simulink model "lineFollowerModel"  (R2020a)
settings: Solver=ode4  StartTime=0.0  StopTime=20  FixedStep=0.0001  RelTol=1e-3
values from neighbouring files (symbols this model uses):
  b = -0.05    [define_constants.m]
  cRoll = 0.1    [define_constants.m]
  g = 9.81    [define_constants.m]
  I_T = 0.1    [define_constants.m]
  I_yy = 5.0000e-05    (= 5e-05)    [define_constants.m]
  K = 0.0089    [define_constants.m]
  L = 2.3E-2    (= 0.023)    [define_constants.m]
  m_T = 1 * mass_scale    [define_constants.m]
  N = 50    [define_constants.m]
  R = 2.2    [define_constants.m]
  row1 = 0.1    [define_constants.m]
  row2 = row1*wheel_ratio_scale    [define_constants.m]
  sX = row1    (= 0.1)    [define_constants.m]
  sY = 0    [define_constants.m]
  Vmax = 12    [define_constants.m]
  W = line_width/2    [define_constants.m]
settings Model: Creator=Amir  LastModifiedBy=matthewterblanche
settings SFSimCC: CustomCodeUndefinedFunction=UseInterfaceOnly

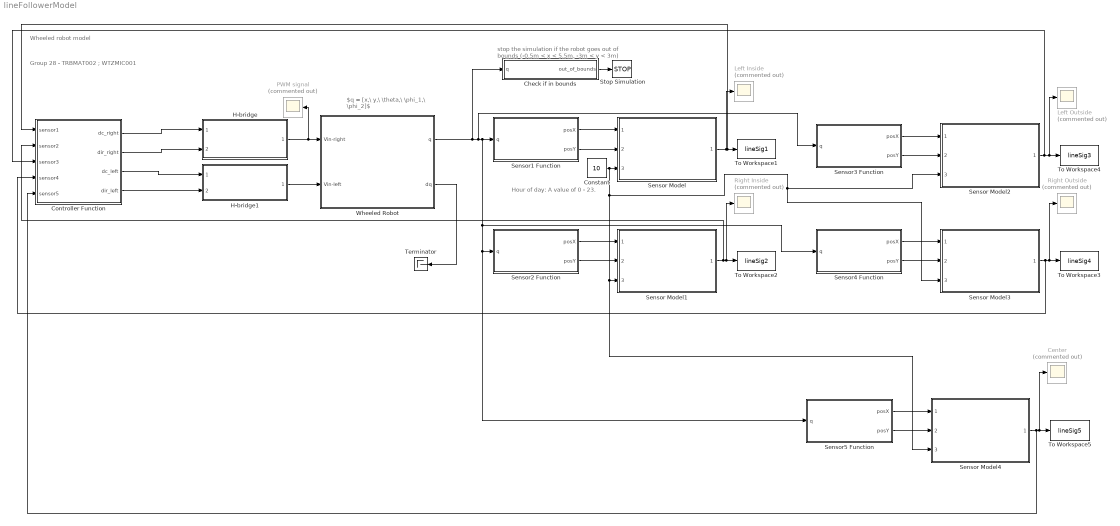
== system lineFollowerModel ==
  note: Group 28 - TRBMAT002 ; WTZMIC001
  note: Hour of day: A value of 0 - 23.
  note: Wheeled robot model
  note: $q = [x,\ y,\ \theta,\ \phi_1,\ \phi_2]$
  note: stop the simulation if the robot goes out of bounds (-0.5m < x < 5.5m, -3m < y < 3m)
  Center : Scope  Commented=on
  Check if in bounds : MATLAB Function  TreatAsAtomicUnit=on
  Constant : Constant  Value=10
  Controller Function : MATLAB Function  TreatAsAtomicUnit=on
  H-bridge : Subsystem  ReferencedSubsystem=H_bridge
  H-bridge1 : Subsystem  ReferencedSubsystem=H_bridge
  Left Inside : Scope  Commented=on
  Left Outside : Scope  Commented=on
  PWM signal : Scope  Commented=on
  Right Inside : Scope  Commented=on
  Right Outside : Scope  Commented=on
  Sensor Model{,1..4} (5 alike) : Subsystem  ReferencedSubsystem=Sensor_Model
  Sensor1 Function : MATLAB Function  TreatAsAtomicUnit=on
  Sensor2 Function : MATLAB Function  TreatAsAtomicUnit=on
  Sensor3 Function : MATLAB Function  TreatAsAtomicUnit=on
  Sensor4 Function : MATLAB Function  TreatAsAtomicUnit=on
  Sensor5 Function : MATLAB Function  TreatAsAtomicUnit=on
  Stop Simulation : Stop
  Terminator : Terminator
  To Workspace1 : ToWorkspace  VariableName=lineSig1  SampleTime=-1
  To Workspace2 : ToWorkspace  VariableName=lineSig2  SampleTime=-1
  To Workspace3 : ToWorkspace  VariableName=lineSig4  SampleTime=-1
  To Workspace4 : ToWorkspace  VariableName=lineSig3  SampleTime=-1
  To Workspace5 : ToWorkspace  VariableName=lineSig5  SampleTime=-1
  Wheeled Robot : Subsystem
  wires:
  H-bridge/1 -> Wheeled Robot/1(Vin-right), PWM signal/1
  H-bridge1/1 -> Wheeled Robot/2(Vin-left)
  Wheeled Robot/2(dq) -> Terminator/1
  Check if in bounds/1(out_of_bounds) -> Stop Simulation/1
  Sensor1 Function/2(posY) -> Sensor Model/2
  Sensor1 Function/1(posX) -> Sensor Model/1
  Sensor Model/1 -> Left Inside/1, Controller Function/1(sensor1), To Workspace1/1
  Sensor2 Function/1(posX) -> Sensor Model1/1
  Sensor2 Function/2(posY) -> Sensor Model1/2
  Sensor Model1/1 -> Controller Function/2(sensor2), Right Inside/1, To Workspace2/1
  Controller Function/1(dc_right) -> H-bridge/1
  Controller Function/2(dir_right) -> H-bridge/2
  Controller Function/3(dc_left) -> H-bridge1/1
  Controller Function/4(dir_left) -> H-bridge1/2
  Sensor4 Function/1(posX) -> Sensor Model3/1
  Sensor4 Function/2(posY) -> Sensor Model3/2
  Constant/1 -> Sensor Model/3, Sensor Model3/3, Sensor Model2/3, Sensor Model4/3, Sensor Model1/3
  Sensor Model2/1 -> Controller Function/3(sensor3), Left Outside/1, To Workspace4/1
  Sensor3 Function/1(posX) -> Sensor Model2/1
  Sensor3 Function/2(posY) -> Sensor Model2/2
  Wheeled Robot/1(q) -> Check if in bounds/1(q), Sensor3 Function/1(q), Sensor4 Function/1(q), Sensor5 Function/1(q), Sensor2 Function/1(q), Sensor1 Function/1(q)
  Sensor Model4/1 -> Controller Function/5(sensor5), Center/1, To Workspace5/1
  Sensor5 Function/1(posX) -> Sensor Model4/1
  Sensor5 Function/2(posY) -> Sensor Model4/2
  Sensor Model3/1 -> Controller Function/4(sensor4), Right Outside/1, To Workspace3/1

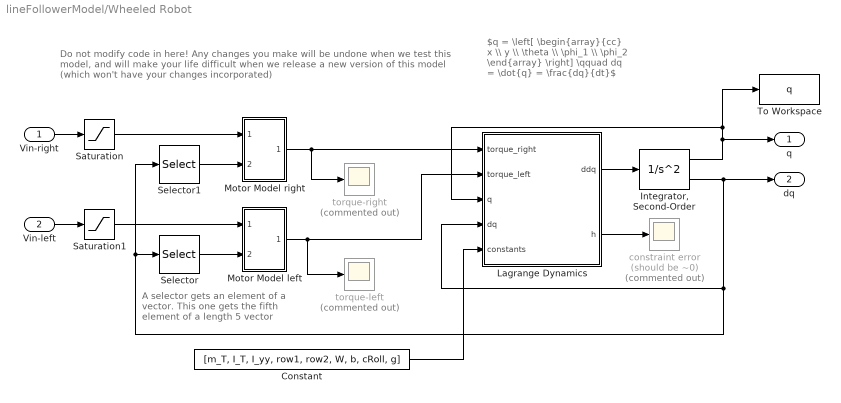
== system lineFollowerModel/Wheeled Robot ==
  note: A selector gets an element of a vector. This one gets the fifth element of a length 5 vector
  note: Do not modify code in here! Any changes you make will be undone when we test this model, and will make your life difficult when we release a new version of this model (which won't have your changes incorporated)
  note: $q = \left[ \begin{array}{cc} x \\ y \\ \theta \\ \phi_1 \\ \phi_2 \end{array} \right] \qquad dq = \dot{q} = \frac{dq}{dt}$
  Vin-right : Inport
  Vin-left : Inport  Port=2
  Constant : Constant  Value=[m_T, I_T, I_yy, row1, row2, W, b, cRoll, g]
  "Integrator, Second-Order" : SecondOrderIntegrator  ICX=[0 0 0 0 0]  ICDXDT=[0 0 0 0 0]
  Lagrange Dynamics : MATLAB Function  TreatAsAtomicUnit=on
  "Motor Model left " : Subsystem
  Motor Model right : Subsystem
  Saturation : Saturate  UpperLimit=Vmax  LowerLimit=-Vmax
  Saturation1 : Saturate  UpperLimit=Vmax  LowerLimit=-Vmax
  Selector : Selector  InputPortWidth=5  IndexOptions=Index vector (dialog)  Indices=[5]  OutputSizes=1
  Selector1 : Selector  InputPortWidth=5  IndexOptions=Index vector (dialog)  Indices=[4]  OutputSizes=1
  To Workspace : ToWorkspace  VariableName=q  SampleTime=0.01
  constraint error (should be ~0) : Scope  Commented=on
  torque-left : Scope  Commented=on
  torque-right : Scope  Commented=on
  q : Outport
  dq : Outport  Port=2
  wires:
  Selector/1 -> "Motor Model left "/2(Omega)
  Selector1/1 -> Motor Model right/2(Omega)
  Motor Model right/1(Tout) -> Lagrange Dynamics/1(torque_right), torque-right/1
  Vin-right/1 -> Saturation/1
  Vin-left/1 -> Saturation1/1
  "Integrator, Second-Order"/1 -> To Workspace/1, Lagrange Dynamics/3(q), q/1
  "Motor Model left "/1(Tout) -> Lagrange Dynamics/2(torque_left), torque-left/1
  "Integrator, Second-Order"/2 -> dq/1, Lagrange Dynamics/4(dq), Selector/1, Selector1/1
  Saturation/1 -> Motor Model right/1(Vin)
  Saturation1/1 -> "Motor Model left "/1(Vin)
  Lagrange Dynamics/1(ddq) -> "Integrator, Second-Order"/1
  Lagrange Dynamics/2(h) -> constraint error (should be ~0)/1
  Constant/1 -> Lagrange Dynamics/5(constants)

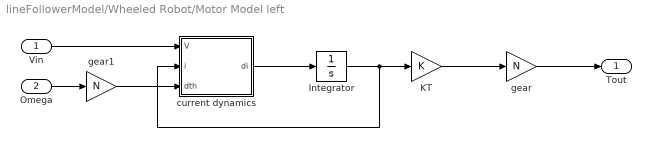
== system lineFollowerModel/Wheeled Robot/Motor Model left  ==
  Vin : Inport
  Omega : Inport  Port=2
  Integrator : Integrator
  KT : Gain  Gain=K
  current dynamics : MATLAB Function  TreatAsAtomicUnit=on
  gear : Gain  Gain=N
  gear1 : Gain  Gain=N
  Tout : Outport  VectorParamsAs1DForOutWhenUnconnected=off
  wires:
  gear1/1 -> current dynamics/3(dth)
  Integrator/1 -> current dynamics/2(i), KT/1
  Omega/1 -> gear1/1
  gear/1 -> Tout/1
  current dynamics/1(di) -> Integrator/1
  KT/1 -> gear/1
  Vin/1 -> current dynamics/1(V)

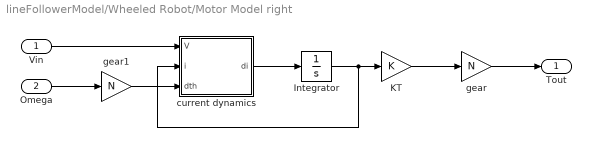
== system lineFollowerModel/Wheeled Robot/Motor Model right ==
  Vin : Inport
  Omega : Inport  Port=2
  Integrator : Integrator
  KT : Gain  Gain=K
  current dynamics : MATLAB Function  TreatAsAtomicUnit=on
  gear : Gain  Gain=N
  gear1 : Gain  Gain=N
  Tout : Outport  VectorParamsAs1DForOutWhenUnconnected=off
  wires:
  Vin/1 -> current dynamics/1(V)
  KT/1 -> gear/1
  current dynamics/1(di) -> Integrator/1
  gear/1 -> Tout/1
  Omega/1 -> gear1/1
  Integrator/1 -> current dynamics/2(i), KT/1
  gear1/1 -> current dynamics/3(dth)

== matlab function lineFollowerModel/Sensor4 Function ==
  data: posX output; q input; sY parameter; sX parameter; posY output
function [posX, posY] = sensor4Position(q, sY, sX)

x = q(1);
y = q(2);
th = q(3);


sX = 0.082;   % Sets sensor just before the front of the robot
sY = -0.082;    % Sets the sensor far right of the line. In the middle of the line and the right side of the robot

posSens_I = [x + sX*cos(th) - sY*sin(th)
    y + sY*cos(th) + sX*sin(th)];

posX = posSens_I(1);
posY = posSens_I(2);

== matlab function lineFollowerModel/Sensor3 Function ==
  data: posX output; q input; sY parameter; sX parameter; posY output
function [posX, posY] = sensor3Position(q, sY, sX)

x = q(1);
y = q(2);
th = q(3);


sX = 0.082;   % Sets sensor just before the front of the robot
sY = 0.085;    % Sets the sensor far left of the line. In the middle of the line and the left side of the robot


posSens_I = [x + sX*cos(th) - sY*sin(th)
    y + sY*cos(th) + sX*sin(th)];

posX = posSens_I(1);
posY = posSens_I(2);

== matlab function lineFollowerModel/Sensor5 Function ==
  data: posX output; q input; sY parameter; sX parameter; posY output
function [posX, posY] = sensor5Position(q, sY, sX)

x = q(1);
y = q(2);
th = q(3);


sX = 0.01;   % Sets sensor at the front of the robot
sY = 0;    % Sets the sensor at the centre of the robot

posSens_I = [x + sX*cos(th) - sY*sin(th)
    y + sY*cos(th) + sX*sin(th)];

posX = posSens_I(1);
posY = posSens_I(2);

== matlab function lineFollowerModel/Wheeled Robot/Motor Model left /current dynamics ==
  data: V input; di output; i input; L parameter; K parameter; R parameter; dth input
function di = dyn(V, i, L, K, R, dth)

di = (V-K*dth-R*i)/L;

== matlab function lineFollowerModel/Wheeled Robot/Lagrange Dynamics ==
  settings: updateMethod=DISCRETE
  data: ddq output size=5; h output size=3; torque_right input; torque_left input; q input; dq input; constants input
%% These dynamics are based on: 
% https://robotics.caltech.edu/~me72/class/DiffDrive2.pdf
% Assume 'd' is 0
function [ddq, h] = dyn(torque_right, torque_left, q, dq, constants)
m_T = constants(1);
I_T = constants(2);
I_yy = constants(3);
row1 = constants(4);
row2 = constants(5);
W = constants(6);
b = constants(7);
cRoll = constants(8);
g = constants(9);

%% Admin
% x = q(1);
% y = q(2);
th = q(3);
% phi1 = q(4);
% phi2 = q(5);

dx = dq(1);
dy = dq(2);
dth = dq(3);
dphi1 = dq(4);
dphi2 = dq(5);


%% Calculate the matrices
% Mass
M = [m_T,   0,   0,    0,    0
       0, m_T,   0,    0,    0
       0,   0, I_T,    0,    0
       0,   0,   0, I_yy,    0
       0,   0,   0,    0, I_yy];

temp = [-sin(th), cos(th), cos(th)
         cos(th), sin(th), sin(th)
               0,     W/2,    -W/2
               0,  - row1,       0
               0,       0,   -row2];

C = transpose(temp);

temp = [ -dth*cos(th), -dth*sin(th), -dth*sin(th)
         -dth*sin(th),  dth*cos(th),  dth*cos(th)
                    0,            0,            0
                    0,            0,            0
                    0,            0,            0];

dC = transpose(temp);

% Input force
T = [0; 0; 0; torque_right + b*dphi1; torque_left + b*dphi2];

% Rolling resistance
vWheel1 = (W*dth)/2 + dx*cos(th) + dy*sin(th);
vWheel2 = dx*cos(th) - (W*dth)/2 + dy*sin(th);
sgnWheel1 = sign(vWheel1);
sgnWheel2 = sign(vWheel2);

F1 = -sgnWheel1*m_T*g*cRoll;
F2 = -sgnWheel2*m_T*g*cRoll;

% input force mapping
Q =  [F1*cos(th) + F2*cos(th)
      F1*sin(th) + F2*sin(th)
          (F1*W)/2 - (F2*W)/2
                            0
                            0];

%% Calculate Lagrange Multipliers
% lambda = -inv(C*inv(M)*transpose(C))*(C*inv(M)*(T+Q) + dC*dq);
lambda = -inv(C*(M\transpose(C)))*(C*(M\(T+Q)) + dC*dq);

h = [                          dy*cos(th) - dx*sin(th)
      (W*dth)/2 - dphi1*row1 + dx*cos(th) + dy*sin(th)
      dx*cos(th) - dphi2*row2 - (W*dth)/2 + dy*sin(th)];


%% Calculate acceleration
ddq = M\(transpose(C)*lambda + T + Q);

end

== matlab function lineFollowerModel/Wheeled Robot/Motor Model right/current dynamics ==
  data: V input; di output; i input; L parameter; K parameter; R parameter; dth input
function di = dyn(V, i, L, K, R, dth)

di = (V - K*dth - R*i)/L;

== matlab function lineFollowerModel/Sensor1 Function ==
  data: posX output; q input; sY parameter; sX parameter; posY output
function [posX, posY] = sensor1Position(q, sY, sX)

x = q(1);
y = q(2);
th = q(3);

sX = 0.1;   % Sets sensor at the front of the robot
sY = 0.019;    % Sets the sensor just to the left of the line


posSens_I = [x + sX*cos(th) - sY*sin(th)
    y + sY*cos(th) + sX*sin(th)];

posX = posSens_I(1);
posY = posSens_I(2);

== matlab function lineFollowerModel/Sensor2 Function ==
  data: posX output; q input; sY parameter; sX parameter; posY output
function [posX, posY] = sensor2Position(q, sY, sX)

x = q(1);
y = q(2);
th = q(3);


sX = 0.1;   % Sets sensor at the front of the robot
sY = -0.024;    % Sets the sensor just to the right of the line

posSens_I = [x + sX*cos(th) - sY*sin(th)
    y + sY*cos(th) + sX*sin(th)];

posX = posSens_I(1);
posY = posSens_I(2);

== matlab function lineFollowerModel/Check if in bounds ==
  data: q input; out_of_bounds output
function out_of_bounds = fcn(q)
x = q(1);
y = q(2);

in_bounds = -0.5 < x && x < 5.5 && -3 < y && y < 3;

out_of_bounds = ~in_bounds;

if out_of_bounds
    disp("Stopping simulation - robot is out of bounds!")
end

== matlab function lineFollowerModel/Controller Function ==
  data: sensor1 input; dc_right output; sensor2 input; dir_right output; dc_left output; dir_left output; sensor3 input; sensor4 input; sensor5 input
function [dc_right,dir_right,dc_left,dir_left] = controller(sensor1, sensor2, sensor3, sensor4, sensor5)

% Persistent variables ensure the value is not reset after every function call

persistent moveLeft;

if isempty(moveLeft)
    moveLeft = 1;
end

persistent moveRight;


if isempty(moveRight)
    moveRight = 1;
end

persistent robotSpeed;

if isempty(robotSpeed)
    robotSpeed = 0.5;
end

persistent calibrating;

if isempty(calibrating)
    calibrating = true;
end


% Mean Value

persistent lineValue;

if isempty(lineValue)
    lineValue = 0.7;
end

persistent threshold;

if isempty(threshold)
    threshold = 0;
end

persistent meanVal;

if isempty(meanVal)
    meanVal = 0;
end

persistent meanArr;

if isempty(meanArr)
    meanArr = zeros(1,100);
end

persistent x;

if isempty(x)
    x = 0;
end

if x < 100
    x = x + 1;
    meanArr(x) = sensor5;
    
    meanVal = mean(meanArr);
    
elseif x == 100
    
    threshold = meanVal*0.72;   % Sets the line threshold
    lineValue = meanVal;        % Sets the mean value of the line
    calibrating = false;
    
    x = x + 1;
    
    
    % Sets unique robot speed for various times of day
    
    if abs(lineValue-0.5243) < 0.001    % Hour 0,1,2,3,4,5,6,21,22,23
        robotSpeed = 0.59;
        
    elseif abs(lineValue-0.5592) < 0.001    % Hour 7
        robotSpeed = 0.59;
        
    elseif abs(lineValue-0.5943) < 0.001    % Hour 20
        robotSpeed = 0.59;
        
    elseif abs(lineValue-0.6290) < 0.001    % Hour 8
        robotSpeed = 0.6;
        
    elseif abs(lineValue-0.6641) < 0.001    % Hour 19
        robotSpeed = 0.59;
        
    elseif abs(lineValue-0.6998) < 0.001    % Hour 9
        robotSpeed = 0.57;
        
    elseif abs(lineValue-0.7700) < 0.001    % Hour 13,14,15,18
        robotSpeed = 0.55;
        
    elseif abs(lineValue-0.8043) < 0.001    % Hour 10,12,17
        robotSpeed = 0.61;
        
    elseif abs(lineValue-0.8396) < 0.001    % Hour 11,16
        robotSpeed = 0.57;
        
    else
        robotSpeed = 0.5;   % Default
    end
end



if calibrating      % Check if robot is in calibrating mode
    
    dc_right = 0;  % Set right motor speed to 0
    dir_right = 0;  % Set right motor direction to 0
    
    dc_left = 0;  % Set left motor speed to 0
    dir_left = 0;  % Set left motor direction to 0
else
    
    
    dc_right = robotSpeed*0.94;  % Set right motor speed to value of robot speed
    dir_right = moveRight;  % Set right motor direction to previously set direction
    
    dc_left = robotSpeed;  % Set left motor speed to value of robot speed
    dir_left = moveLeft;  % Set left motor direction to previously set direction
    
    
    
    % Move robot to stay on line
    
    if sensor1 > threshold    % Turn robot left if inner left sensor (S1) touches line
        
        dc_left = dc_left*0.5;  % Set left wheel speed to 50% of top speed
        
    end
    
    if sensor3 > threshold    % Turn robot sharp left if outer left sensor (S3) touches line
        
        % Set right wheel to go forward and left wheel to go in reverse
        moveRight = 1;
        dir_right = moveRight;
        moveLeft = 1;
        dir_left = -1;
        
    end
    
    
    if sensor2 > threshold     % Turn robot right if inner right sensor (S2) touches line
        
        dc_right = dc_right*0.5;  % Set right wheel speed to 50% of top speed
        
        
    end
    
    if  sensor4 > threshold    % Turn robot sharp right if outer right sensor (S4) touches line
        
        
        % Set left wheel to go forward and right wheel to go in reverse
        moveLeft = 1;
        dir_left = moveLeft;
        moveRight = 1;
        dir_right = -1;
        
        
    end
    
    
    
    % Stop robot at double line
    
    if (sensor1 > threshold*0.95  && sensor2 > threshold*0.95  ) || (sensor3 > threshold*0.95  && sensor4 > threshold*0.95 )
        
        % If both inner sensors (S1 & S2) touch the line
        % or both outer sensors (S3 & S4) touch the line then stop the robot
        
        robotSpeed = 0;
        
        dc_right = robotSpeed;  % Stop right motor
        dc_left =robotSpeed;  % Stop right motor
        
        dir_left = robotSpeed;  % Stop right motor
        dir_right = robotSpeed;  % Stop right motor
        
        
        
    end
    
end
